simulink model "qdrdac_newphscrct"  (R2012b)
settings: Solver=ode45  StartTime=0.0  StopTime=22000  RelTol=1e-3
undefined symbols (not defined in the file or in its folder): pfb_coeff_gen_calc, sfp
libraries: xbsIndex_r4 x3696, casper_library_misc x76, xps_library x14, casper_library_delays x12, maddogLibrary x4, simulink x2
(part 9 of 37)

== system qdrdac_newphscrct/pfb_fir1 ==
  sync : Inport
  pol1_in1 : Inport  Port=2
  pol1_in2 : Inport  Port=3
  pol1_in3 : Inport  Port=4
  pol1_in4 : Inport  Port=5
  pol1_in1_coeffs : Subsystem  AncestorBlock=casper_library_pfbs/pfb_coeff_gen  mask(pfb_coeff_gen){PFBSize=9, CoeffBitWidth=18, TotalTaps=4, CoeffDistMem=off, WindowType=hamming, bram_latency=2, n_inputs=2, nput=0, fwidth=1, debug_mode=off, fan_latency=1}
      mask prompts: PFBSize "Size of PFB: (2^? pnts)"; CoeffBitWidth "Bitwidth of Coefficients:"; TotalTaps "Total Number of Taps:"; CoeffDistMem "Implement Coeff Gen in Distributed Memory"; WindowType "Windowing Function:"; bram_latency "BRAM Latency"; n_inputs "Number of Simultaneous Inputs: (2^?)"; nput "This is input number:"; fwidth "Bin Width (normal=1)"; debug_mode "Debug mode - coeffs are a [1:pfb_size*taps] ramp."; fan_latency "Fanout latency"
      mask init:
      | pfb_coeff_gen_init(gcb, ...
      |     'PFBSize', PFBSize, ...
      |     'CoeffBitWidth', CoeffBitWidth, ...
      |     'TotalTaps', TotalTaps, ...
      |     'CoeffDistMem', CoeffDistMem, ...
      |     'WindowType', WindowType, ...
      |     'bram_latency', bram_latency, ...
      |     'n_inputs', n_inputs, ...
      |     'nput', nput, ...
      |     'fwidth', fwidth, ...
      |     'fan_latency', fan_latency, ...
      |     'debug_mode', debug_mode);
      settings: AttributesFormatString=|
      | PFBSize=9, n_inputs=2,
      | taps=4, input=0
  pol1_in1_first_tap : Subsystem  AncestorBlock=casper_library_pfbs/first_tap  mask(first_tap){PFBSize=9, CoeffBitWidth=18, TotalTaps=4, BitWidthIn=12, WindowType=hamming, mult_latency=2, bram_latency=2, n_inputs=2, fwidth=1, use_hdl=on, use_embedded=off}
      mask prompts: PFBSize "Size of PFB: (2^? pnts)"; CoeffBitWidth "Bitwidth of Coefficients:"; TotalTaps "Total Number of Taps:"; BitWidthIn "Input Bitwidth:"; WindowType "Windowing Function:"; mult_latency "Mult Latency"; bram_latency "BRAM Latency"; n_inputs "Number of Simultaneous Inputs: (2^?)"; fwidth "Bit Width (normal=1)"; use_hdl "Use behavioral HDL for multlipliers"; use_embedded "Use embedded multipliers"
      mask init:
      | first_tap_init(gcb,...
      |     'PFBSize', PFBSize,...
      |     'CoeffBitWidth', CoeffBitWidth,...
      |     'TotalTaps', TotalTaps,...
      |     'BitWidthIn', BitWidthIn,...
      |     'WindowType', WindowType,...
      |     'mult_latency', mult_latency,...
      |     'bram_latency', bram_latency,...
      |     'n_inputs', n_inputs,...
      |     'fwidth', fwidth,...
      |     'use_hdl', use_hdl,...
      |     'use_embedded', use_embedded);
      settings: AttributesFormatString=taps=4
      mask TypeOptions WindowType: bartlett | barthannwin | blackman | blackmanharris | bohamwin | chebwin | flattopwin | gausswin | hamming | hann | kaiser | nuttallwin | parzenwin | rectwin | tukeywin | triang
      mask Callback use_hdl:
      | use_hdl = get_param(gcb,'use_hdl');
      | if( strcmp(use_hdl,'on')),
      |     set_param(gcb, 'use_embedded','off');
      |     set_param(gcb, 'MaskVisibilities',{'on','on','on','on','on','on','on','on','on','on','off'});
      | else,
      |     set_param(gcb, 'MaskVisibilities',{'on','on','on','on','on','on','on','on','on','on','on'});
      | end
  pol1_in1_last_tap : Subsystem  AncestorBlock=casper_library_pfbs/last_tap  mask(last_tap){TotalTaps=4, BitWidthIn=12, BitWidthOut=18, CoeffBitWidth=18, add_latency=1, mult_latency=2, quantization=Truncate, use_hdl=on, use_embedded=off}
      mask prompts: TotalTaps "Total Number of Taps:"; BitWidthIn "Input Bitwidth:"; BitWidthOut "Output Bitwidth:"; CoeffBitWidth "Coeff Bitwidth:"; add_latency "Add Latency"; mult_latency "Mult Latency"; quantization "Quantization Behavior"; use_hdl "Use behavioral HDL for multlipliers"; use_embedded "Use embedded multipliers"
      mask init:
      | last_tap_init(gcb,...
      |     'TotalTaps', TotalTaps,...
      |     'BitWidthIn', BitWidthIn,...
      |     'BitWidthOut', BitWidthOut,...
      |     'CoeffBitWidth', CoeffBitWidth,...
      |     'add_latency', add_latency,...
      |     'mult_latency', mult_latency,...
      |     'quantization', quantization,...
      |     'use_hdl', use_hdl,...
      |     'use_embedded', use_embedded);
      settings: AttributesFormatString=taps=4
      mask TypeOptions quantization: Truncate | Round  (unbiased: +/- Inf) | Round  (unbiased: Even Values)
      mask Callback use_hdl:
      | use_hdl = get_param(gcb,'use_hdl');
      | if( strcmp(use_hdl,'on')),
      |     set_param(gcb, 'use_embedded','off');
      |     set_param(gcb, 'MaskVisibilities',{'on','on','on','on','on','on','on','on','off'});
      | else,
      |     set_param(gcb, 'MaskVisibilities',{'on','on','on','on','on','on','on','on','on'});
      | end
  pol1_in1_tap2 : Subsystem  AncestorBlock=casper_library_pfbs/tap  mask(tap){mult_latency=2, coeff_width=18, coeff_frac_width=17, delay=128, data_width=12, bram_latency=2, use_hdl=on, use_embedded=off}
      mask prompts: mult_latency "Multiplier Latency"; coeff_width "Coefficient Bit Width In"; coeff_frac_width "Coefficient Fractional Bits"; delay "Data/Sync Delay"; data_width "Data Bit Width In"; bram_latency "BRAM Latency"; use_hdl "Use behavioral HDL for multlipliers"; use_embedded "Use embedded multipliers"
      mask init:
      | use_hdl = get_param(gcb,'use_hdl');
      | use_embedded = get_param(gcb,'use_embedded');
      | set_param(gcb,'LinkStatus','inactive');
      | 
      | set_param([gcb,'/Mult'],'use_embedded',use_embedded);
      | set_param([gcb,'/Mult'],'use_behavioral_HDL',use_hdl);
      | set_param([gcb,'/Mult1'],'use_embedded',use_embedded);
      | set_param([gcb,'/Mult1'],'use_behavioral_HDL',use_hdl);
      mask Callback use_hdl:
      | use_hdl = get_param(gcb,'use_hdl');
      | if( strcmp(use_hdl,'on')),
      |     set_param(gcb, 'use_embedded','off');
      |     set_param(gcb, 'MaskVisibilities',{'on','on','on','on','on','on','on','off'});
      | else,
      |     set_param(gcb, 'MaskVisibilities',{'on','on','on','on','on','on','on','on'});
      | end
  pol1_in1_tap3 : Subsystem  AncestorBlock=casper_library_pfbs/tap  mask(tap){mult_latency=2, coeff_width=18, coeff_frac_width=17, delay=128, data_width=12, bram_latency=2, use_hdl=on, use_embedded=off}
      mask prompts: mult_latency "Multiplier Latency"; coeff_width "Coefficient Bit Width In"; coeff_frac_width "Coefficient Fractional Bits"; delay "Data/Sync Delay"; data_width "Data Bit Width In"; bram_latency "BRAM Latency"; use_hdl "Use behavioral HDL for multlipliers"; use_embedded "Use embedded multipliers"
      mask init: same as qdrdac_newphscrct/pfb_fir1/pol1_in1_tap2
      mask Callback use_hdl:
      | use_hdl = get_param(gcb,'use_hdl');
      | if( strcmp(use_hdl,'on')),
      |     set_param(gcb, 'use_embedded','off');
      |     set_param(gcb, 'MaskVisibilities',{'on','on','on','on','on','on','on','off'});
      | else,
      |     set_param(gcb, 'MaskVisibilities',{'on','on','on','on','on','on','on','on'});
      | end
  pol1_in2_coeffs : Subsystem  AncestorBlock=casper_library_pfbs/pfb_coeff_gen  mask(pfb_coeff_gen){PFBSize=9, CoeffBitWidth=18, TotalTaps=4, CoeffDistMem=off, WindowType=hamming, bram_latency=2, n_inputs=2, nput=1, fwidth=1, debug_mode=off, fan_latency=1}
      mask prompts: PFBSize "Size of PFB: (2^? pnts)"; CoeffBitWidth "Bitwidth of Coefficients:"; TotalTaps "Total Number of Taps:"; CoeffDistMem "Implement Coeff Gen in Distributed Memory"; WindowType "Windowing Function:"; bram_latency "BRAM Latency"; n_inputs "Number of Simultaneous Inputs: (2^?)"; nput "This is input number:"; fwidth "Bin Width (normal=1)"; debug_mode "Debug mode - coeffs are a [1:pfb_size*taps] ramp."; fan_latency "Fanout latency"
      mask init: same as qdrdac_newphscrct/pfb_fir1/pol1_in1_coeffs
      settings: AttributesFormatString=|
      | PFBSize=9, n_inputs=2,
      | taps=4, input=1
  pol1_in2_first_tap : Subsystem  AncestorBlock=casper_library_pfbs/first_tap  mask(first_tap){PFBSize=9, CoeffBitWidth=18, TotalTaps=4, BitWidthIn=12, WindowType=hamming, mult_latency=2, bram_latency=2, n_inputs=2, fwidth=1, use_hdl=on, use_embedded=off}
      mask prompts: PFBSize "Size of PFB: (2^? pnts)"; CoeffBitWidth "Bitwidth of Coefficients:"; TotalTaps "Total Number of Taps:"; BitWidthIn "Input Bitwidth:"; WindowType "Windowing Function:"; mult_latency "Mult Latency"; bram_latency "BRAM Latency"; n_inputs "Number of Simultaneous Inputs: (2^?)"; fwidth "Bit Width (normal=1)"; use_hdl "Use behavioral HDL for multlipliers"; use_embedded "Use embedded multipliers"
      mask init: same as qdrdac_newphscrct/pfb_fir1/pol1_in1_first_tap
      settings: AttributesFormatString=taps=4
      mask TypeOptions WindowType: bartlett | barthannwin | blackman | blackmanharris | bohamwin | chebwin | flattopwin | gausswin | hamming | hann | kaiser | nuttallwin | parzenwin | rectwin | tukeywin | triang
      mask Callback use_hdl:
      | use_hdl = get_param(gcb,'use_hdl');
      | if( strcmp(use_hdl,'on')),
      |     set_param(gcb, 'use_embedded','off');
      |     set_param(gcb, 'MaskVisibilities',{'on','on','on','on','on','on','on','on','on','on','off'});
      | else,
      |     set_param(gcb, 'MaskVisibilities',{'on','on','on','on','on','on','on','on','on','on','on'});
      | end
  pol1_in2_last_tap : Subsystem  AncestorBlock=casper_library_pfbs/last_tap  mask(last_tap){TotalTaps=4, BitWidthIn=12, BitWidthOut=18, CoeffBitWidth=18, add_latency=1, mult_latency=2, quantization=Truncate, use_hdl=on, use_embedded=off}
      mask prompts: TotalTaps "Total Number of Taps:"; BitWidthIn "Input Bitwidth:"; BitWidthOut "Output Bitwidth:"; CoeffBitWidth "Coeff Bitwidth:"; add_latency "Add Latency"; mult_latency "Mult Latency"; quantization "Quantization Behavior"; use_hdl "Use behavioral HDL for multlipliers"; use_embedded "Use embedded multipliers"
      mask init: same as qdrdac_newphscrct/pfb_fir1/pol1_in1_last_tap
      settings: AttributesFormatString=taps=4
      mask TypeOptions quantization: Truncate | Round  (unbiased: +/- Inf) | Round  (unbiased: Even Values)
      mask Callback use_hdl:
      | use_hdl = get_param(gcb,'use_hdl');
      | if( strcmp(use_hdl,'on')),
      |     set_param(gcb, 'use_embedded','off');
      |     set_param(gcb, 'MaskVisibilities',{'on','on','on','on','on','on','on','on','off'});
      | else,
      |     set_param(gcb, 'MaskVisibilities',{'on','on','on','on','on','on','on','on','on'});
      | end
  pol1_in2_tap2 : Subsystem  AncestorBlock=casper_library_pfbs/tap  mask(tap){mult_latency=2, coeff_width=18, coeff_frac_width=17, delay=128, data_width=12, bram_latency=2, use_hdl=on, use_embedded=off}
      mask prompts: mult_latency "Multiplier Latency"; coeff_width "Coefficient Bit Width In"; coeff_frac_width "Coefficient Fractional Bits"; delay "Data/Sync Delay"; data_width "Data Bit Width In"; bram_latency "BRAM Latency"; use_hdl "Use behavioral HDL for multlipliers"; use_embedded "Use embedded multipliers"
      mask init: same as qdrdac_newphscrct/pfb_fir1/pol1_in1_tap2
      mask Callback use_hdl:
      | use_hdl = get_param(gcb,'use_hdl');
      | if( strcmp(use_hdl,'on')),
      |     set_param(gcb, 'use_embedded','off');
      |     set_param(gcb, 'MaskVisibilities',{'on','on','on','on','on','on','on','off'});
      | else,
      |     set_param(gcb, 'MaskVisibilities',{'on','on','on','on','on','on','on','on'});
      | end
  pol1_in2_tap3 : Subsystem  AncestorBlock=casper_library_pfbs/tap  mask(tap){mult_latency=2, coeff_width=18, coeff_frac_width=17, delay=128, data_width=12, bram_latency=2, use_hdl=on, use_embedded=off}
      mask prompts: mult_latency "Multiplier Latency"; coeff_width "Coefficient Bit Width In"; coeff_frac_width "Coefficient Fractional Bits"; delay "Data/Sync Delay"; data_width "Data Bit Width In"; bram_latency "BRAM Latency"; use_hdl "Use behavioral HDL for multlipliers"; use_embedded "Use embedded multipliers"
      mask init: same as qdrdac_newphscrct/pfb_fir1/pol1_in1_tap2
      mask Callback use_hdl:
      | use_hdl = get_param(gcb,'use_hdl');
      | if( strcmp(use_hdl,'on')),
      |     set_param(gcb, 'use_embedded','off');
      |     set_param(gcb, 'MaskVisibilities',{'on','on','on','on','on','on','on','off'});
      | else,
      |     set_param(gcb, 'MaskVisibilities',{'on','on','on','on','on','on','on','on'});
      | end
  pol1_in3_coeffs : Subsystem  AncestorBlock=casper_library_pfbs/pfb_coeff_gen  mask(pfb_coeff_gen){PFBSize=9, CoeffBitWidth=18, TotalTaps=4, CoeffDistMem=off, WindowType=hamming, bram_latency=2, n_inputs=2, nput=2, fwidth=1, debug_mode=off, fan_latency=1}
      mask prompts: PFBSize "Size of PFB: (2^? pnts)"; CoeffBitWidth "Bitwidth of Coefficients:"; TotalTaps "Total Number of Taps:"; CoeffDistMem "Implement Coeff Gen in Distributed Memory"; WindowType "Windowing Function:"; bram_latency "BRAM Latency"; n_inputs "Number of Simultaneous Inputs: (2^?)"; nput "This is input number:"; fwidth "Bin Width (normal=1)"; debug_mode "Debug mode - coeffs are a [1:pfb_size*taps] ramp."; fan_latency "Fanout latency"
      mask init: same as qdrdac_newphscrct/pfb_fir1/pol1_in1_coeffs
      settings: AttributesFormatString=|
      | PFBSize=9, n_inputs=2,
      | taps=4, input=2
  pol1_in3_first_tap : Subsystem  AncestorBlock=casper_library_pfbs/first_tap  mask(first_tap){PFBSize=9, CoeffBitWidth=18, TotalTaps=4, BitWidthIn=12, WindowType=hamming, mult_latency=2, bram_latency=2, n_inputs=2, fwidth=1, use_hdl=on, use_embedded=off}
      mask prompts: PFBSize "Size of PFB: (2^? pnts)"; CoeffBitWidth "Bitwidth of Coefficients:"; TotalTaps "Total Number of Taps:"; BitWidthIn "Input Bitwidth:"; WindowType "Windowing Function:"; mult_latency "Mult Latency"; bram_latency "BRAM Latency"; n_inputs "Number of Simultaneous Inputs: (2^?)"; fwidth "Bit Width (normal=1)"; use_hdl "Use behavioral HDL for multlipliers"; use_embedded "Use embedded multipliers"
      mask init: same as qdrdac_newphscrct/pfb_fir1/pol1_in1_first_tap
      settings: AttributesFormatString=taps=4
      mask TypeOptions WindowType: bartlett | barthannwin | blackman | blackmanharris | bohamwin | chebwin | flattopwin | gausswin | hamming | hann | kaiser | nuttallwin | parzenwin | rectwin | tukeywin | triang
      mask Callback use_hdl:
      | use_hdl = get_param(gcb,'use_hdl');
      | if( strcmp(use_hdl,'on')),
      |     set_param(gcb, 'use_embedded','off');
      |     set_param(gcb, 'MaskVisibilities',{'on','on','on','on','on','on','on','on','on','on','off'});
      | else,
      |     set_param(gcb, 'MaskVisibilities',{'on','on','on','on','on','on','on','on','on','on','on'});
      | end
  pol1_in3_last_tap : Subsystem  AncestorBlock=casper_library_pfbs/last_tap  mask(last_tap){TotalTaps=4, BitWidthIn=12, BitWidthOut=18, CoeffBitWidth=18, add_latency=1, mult_latency=2, quantization=Truncate, use_hdl=on, use_embedded=off}
      mask prompts: TotalTaps "Total Number of Taps:"; BitWidthIn "Input Bitwidth:"; BitWidthOut "Output Bitwidth:"; CoeffBitWidth "Coeff Bitwidth:"; add_latency "Add Latency"; mult_latency "Mult Latency"; quantization "Quantization Behavior"; use_hdl "Use behavioral HDL for multlipliers"; use_embedded "Use embedded multipliers"
      mask init: same as qdrdac_newphscrct/pfb_fir1/pol1_in1_last_tap
      settings: AttributesFormatString=taps=4
      mask TypeOptions quantization: Truncate | Round  (unbiased: +/- Inf) | Round  (unbiased: Even Values)
      mask Callback use_hdl:
      | use_hdl = get_param(gcb,'use_hdl');
      | if( strcmp(use_hdl,'on')),
      |     set_param(gcb, 'use_embedded','off');
      |     set_param(gcb, 'MaskVisibilities',{'on','on','on','on','on','on','on','on','off'});
      | else,
      |     set_param(gcb, 'MaskVisibilities',{'on','on','on','on','on','on','on','on','on'});
      | end
  pol1_in3_tap2 : Subsystem  AncestorBlock=casper_library_pfbs/tap  mask(tap){mult_latency=2, coeff_width=18, coeff_frac_width=17, delay=128, data_width=12, bram_latency=2, use_hdl=on, use_embedded=off}
      mask prompts: mult_latency "Multiplier Latency"; coeff_width "Coefficient Bit Width In"; coeff_frac_width "Coefficient Fractional Bits"; delay "Data/Sync Delay"; data_width "Data Bit Width In"; bram_latency "BRAM Latency"; use_hdl "Use behavioral HDL for multlipliers"; use_embedded "Use embedded multipliers"
      mask init: same as qdrdac_newphscrct/pfb_fir1/pol1_in1_tap2
      mask Callback use_hdl:
      | use_hdl = get_param(gcb,'use_hdl');
      | if( strcmp(use_hdl,'on')),
      |     set_param(gcb, 'use_embedded','off');
      |     set_param(gcb, 'MaskVisibilities',{'on','on','on','on','on','on','on','off'});
      | else,
      |     set_param(gcb, 'MaskVisibilities',{'on','on','on','on','on','on','on','on'});
      | end
  pol1_in3_tap3 : Subsystem  AncestorBlock=casper_library_pfbs/tap  mask(tap){mult_latency=2, coeff_width=18, coeff_frac_width=17, delay=128, data_width=12, bram_latency=2, use_hdl=on, use_embedded=off}
      mask prompts: mult_latency "Multiplier Latency"; coeff_width "Coefficient Bit Width In"; coeff_frac_width "Coefficient Fractional Bits"; delay "Data/Sync Delay"; data_width "Data Bit Width In"; bram_latency "BRAM Latency"; use_hdl "Use behavioral HDL for multlipliers"; use_embedded "Use embedded multipliers"
      mask init: same as qdrdac_newphscrct/pfb_fir1/pol1_in1_tap2
      mask Callback use_hdl:
      | use_hdl = get_param(gcb,'use_hdl');
      | if( strcmp(use_hdl,'on')),
      |     set_param(gcb, 'use_embedded','off');
      |     set_param(gcb, 'MaskVisibilities',{'on','on','on','on','on','on','on','off'});
      | else,
      |     set_param(gcb, 'MaskVisibilities',{'on','on','on','on','on','on','on','on'});
      | end
  pol1_in4_coeffs : Subsystem  AncestorBlock=casper_library_pfbs/pfb_coeff_gen  mask(pfb_coeff_gen){PFBSize=9, CoeffBitWidth=18, TotalTaps=4, CoeffDistMem=off, WindowType=hamming, bram_latency=2, n_inputs=2, nput=3, fwidth=1, debug_mode=off, fan_latency=1}
      mask prompts: PFBSize "Size of PFB: (2^? pnts)"; CoeffBitWidth "Bitwidth of Coefficients:"; TotalTaps "Total Number of Taps:"; CoeffDistMem "Implement Coeff Gen in Distributed Memory"; WindowType "Windowing Function:"; bram_latency "BRAM Latency"; n_inputs "Number of Simultaneous Inputs: (2^?)"; nput "This is input number:"; fwidth "Bin Width (normal=1)"; debug_mode "Debug mode - coeffs are a [1:pfb_size*taps] ramp."; fan_latency "Fanout latency"
      mask init: same as qdrdac_newphscrct/pfb_fir1/pol1_in1_coeffs
      settings: AttributesFormatString=|
      | PFBSize=9, n_inputs=2,
      | taps=4, input=3
  pol1_in4_first_tap : Subsystem  AncestorBlock=casper_library_pfbs/first_tap  mask(first_tap){PFBSize=9, CoeffBitWidth=18, TotalTaps=4, BitWidthIn=12, WindowType=hamming, mult_latency=2, bram_latency=2, n_inputs=2, fwidth=1, use_hdl=on, use_embedded=off}
      mask prompts: PFBSize "Size of PFB: (2^? pnts)"; CoeffBitWidth "Bitwidth of Coefficients:"; TotalTaps "Total Number of Taps:"; BitWidthIn "Input Bitwidth:"; WindowType "Windowing Function:"; mult_latency "Mult Latency"; bram_latency "BRAM Latency"; n_inputs "Number of Simultaneous Inputs: (2^?)"; fwidth "Bit Width (normal=1)"; use_hdl "Use behavioral HDL for multlipliers"; use_embedded "Use embedded multipliers"
      mask init: same as qdrdac_newphscrct/pfb_fir1/pol1_in1_first_tap
      settings: AttributesFormatString=taps=4
      mask TypeOptions WindowType: bartlett | barthannwin | blackman | blackmanharris | bohamwin | chebwin | flattopwin | gausswin | hamming | hann | kaiser | nuttallwin | parzenwin | rectwin | tukeywin | triang
      mask Callback use_hdl:
      | use_hdl = get_param(gcb,'use_hdl');
      | if( strcmp(use_hdl,'on')),
      |     set_param(gcb, 'use_embedded','off');
      |     set_param(gcb, 'MaskVisibilities',{'on','on','on','on','on','on','on','on','on','on','off'});
      | else,
      |     set_param(gcb, 'MaskVisibilities',{'on','on','on','on','on','on','on','on','on','on','on'});
      | end
  pol1_in4_last_tap : Subsystem  AncestorBlock=casper_library_pfbs/last_tap  mask(last_tap){TotalTaps=4, BitWidthIn=12, BitWidthOut=18, CoeffBitWidth=18, add_latency=1, mult_latency=2, quantization=Truncate, use_hdl=on, use_embedded=off}
      mask prompts: TotalTaps "Total Number of Taps:"; BitWidthIn "Input Bitwidth:"; BitWidthOut "Output Bitwidth:"; CoeffBitWidth "Coeff Bitwidth:"; add_latency "Add Latency"; mult_latency "Mult Latency"; quantization "Quantization Behavior"; use_hdl "Use behavioral HDL for multlipliers"; use_embedded "Use embedded multipliers"
      mask init: same as qdrdac_newphscrct/pfb_fir1/pol1_in1_last_tap
      settings: AttributesFormatString=taps=4
      mask TypeOptions quantization: Truncate | Round  (unbiased: +/- Inf) | Round  (unbiased: Even Values)
      mask Callback use_hdl:
      | use_hdl = get_param(gcb,'use_hdl');
      | if( strcmp(use_hdl,'on')),
      |     set_param(gcb, 'use_embedded','off');
      |     set_param(gcb, 'MaskVisibilities',{'on','on','on','on','on','on','on','on','off'});
      | else,
      |     set_param(gcb, 'MaskVisibilities',{'on','on','on','on','on','on','on','on','on'});
      | end
  pol1_in4_tap2 : Subsystem  AncestorBlock=casper_library_pfbs/tap  mask(tap){mult_latency=2, coeff_width=18, coeff_frac_width=17, delay=128, data_width=12, bram_latency=2, use_hdl=on, use_embedded=off}
      mask prompts: mult_latency "Multiplier Latency"; coeff_width "Coefficient Bit Width In"; coeff_frac_width "Coefficient Fractional Bits"; delay "Data/Sync Delay"; data_width "Data Bit Width In"; bram_latency "BRAM Latency"; use_hdl "Use behavioral HDL for multlipliers"; use_embedded "Use embedded multipliers"
      mask init: same as qdrdac_newphscrct/pfb_fir1/pol1_in1_tap2
      mask Callback use_hdl:
      | use_hdl = get_param(gcb,'use_hdl');
      | if( strcmp(use_hdl,'on')),
      |     set_param(gcb, 'use_embedded','off');
      |     set_param(gcb, 'MaskVisibilities',{'on','on','on','on','on','on','on','off'});
      | else,
      |     set_param(gcb, 'MaskVisibilities',{'on','on','on','on','on','on','on','on'});
      | end
  pol1_in4_tap3 : Subsystem  AncestorBlock=casper_library_pfbs/tap  mask(tap){mult_latency=2, coeff_width=18, coeff_frac_width=17, delay=128, data_width=12, bram_latency=2, use_hdl=on, use_embedded=off}
      mask prompts: mult_latency "Multiplier Latency"; coeff_width "Coefficient Bit Width In"; coeff_frac_width "Coefficient Fractional Bits"; delay "Data/Sync Delay"; data_width "Data Bit Width In"; bram_latency "BRAM Latency"; use_hdl "Use behavioral HDL for multlipliers"; use_embedded "Use embedded multipliers"
      mask init: same as qdrdac_newphscrct/pfb_fir1/pol1_in1_tap2
      mask Callback use_hdl:
      | use_hdl = get_param(gcb,'use_hdl');
      | if( strcmp(use_hdl,'on')),
      |     set_param(gcb, 'use_embedded','off');
      |     set_param(gcb, 'MaskVisibilities',{'on','on','on','on','on','on','on','off'});
      | else,
      |     set_param(gcb, 'MaskVisibilities',{'on','on','on','on','on','on','on','on'});
      | end
  sync_out : Outport
  pol1_out1 : Outport  Port=2
  pol1_out2 : Outport  Port=3
  pol1_out3 : Outport  Port=4
  pol1_out4 : Outport  Port=5
  wires:
  pol1_in1/1 -> pol1_in1_coeffs/1(din)
  sync/1 -> pol1_in1_coeffs/2(sync), pol1_in2_coeffs/2(sync), pol1_in3_coeffs/2(sync), pol1_in4_coeffs/2(sync)
  pol1_in1_coeffs/1(dout) -> pol1_in1_first_tap/1(din)
  pol1_in1_coeffs/2(sync_out) -> pol1_in1_first_tap/2(sync), pol1_in2_first_tap/2(sync), pol1_in3_first_tap/2(sync), pol1_in4_first_tap/2(sync)
  pol1_in1_coeffs/3(coeff) -> pol1_in1_first_tap/3(coeffs)
  pol1_in1_first_tap/1(dout) -> pol1_in1_tap2/1(din)
  pol1_in1_first_tap/2(sync_out) -> pol1_in1_tap2/2(sync)
  pol1_in1_first_tap/3(coeff_out) -> pol1_in1_tap2/3(coeff)
  pol1_in1_first_tap/4(taps_out) -> pol1_in1_tap2/4(taps)
  pol1_in1_tap2/1(dout) -> pol1_in1_tap3/1(din)
  pol1_in1_tap2/2(sync_out) -> pol1_in1_tap3/2(sync)
  pol1_in1_tap2/3(coeff_out) -> pol1_in1_tap3/3(coeff)
  pol1_in1_tap2/4(taps_out) -> pol1_in1_tap3/4(taps)
  pol1_in1_tap3/1(dout) -> pol1_in1_last_tap/1(din)
  pol1_in1_tap3/2(sync_out) -> pol1_in1_last_tap/2(sync)
  pol1_in1_tap3/3(coeff_out) -> pol1_in1_last_tap/3(coeff)
  pol1_in1_tap3/4(taps_out) -> pol1_in1_last_tap/4(taps)
  pol1_in1_last_tap/1(dout) -> pol1_out1/1
  pol1_in1_last_tap/2(sync_out) -> sync_out/1
  pol1_in2/1 -> pol1_in2_coeffs/1(din)
  pol1_in2_coeffs/1(dout) -> pol1_in2_first_tap/1(din)
  pol1_in2_coeffs/3(coeff) -> pol1_in2_first_tap/3(coeffs)
  pol1_in2_first_tap/1(dout) -> pol1_in2_tap2/1(din)
  pol1_in2_first_tap/2(sync_out) -> pol1_in2_tap2/2(sync)
  pol1_in2_first_tap/3(coeff_out) -> pol1_in2_tap2/3(coeff)
  pol1_in2_first_tap/4(taps_out) -> pol1_in2_tap2/4(taps)
  pol1_in2_tap2/1(dout) -> pol1_in2_tap3/1(din)
  pol1_in2_tap2/2(sync_out) -> pol1_in2_tap3/2(sync)
  pol1_in2_tap2/3(coeff_out) -> pol1_in2_tap3/3(coeff)
  pol1_in2_tap2/4(taps_out) -> pol1_in2_tap3/4(taps)
  pol1_in2_tap3/1(dout) -> pol1_in2_last_tap/1(din)
  pol1_in2_tap3/2(sync_out) -> pol1_in2_last_tap/2(sync)
  pol1_in2_tap3/3(coeff_out) -> pol1_in2_last_tap/3(coeff)
  pol1_in2_tap3/4(taps_out) -> pol1_in2_last_tap/4(taps)
  pol1_in2_last_tap/1(dout) -> pol1_out2/1
  pol1_in3/1 -> pol1_in3_coeffs/1(din)
  pol1_in3_coeffs/1(dout) -> pol1_in3_first_tap/1(din)
  pol1_in3_coeffs/3(coeff) -> pol1_in3_first_tap/3(coeffs)
  pol1_in3_first_tap/1(dout) -> pol1_in3_tap2/1(din)
  pol1_in3_first_tap/2(sync_out) -> pol1_in3_tap2/2(sync)
  pol1_in3_first_tap/3(coeff_out) -> pol1_in3_tap2/3(coeff)
  pol1_in3_first_tap/4(taps_out) -> pol1_in3_tap2/4(taps)
  pol1_in3_tap2/1(dout) -> pol1_in3_tap3/1(din)
  pol1_in3_tap2/2(sync_out) -> pol1_in3_tap3/2(sync)
  pol1_in3_tap2/3(coeff_out) -> pol1_in3_tap3/3(coeff)
  pol1_in3_tap2/4(taps_out) -> pol1_in3_tap3/4(taps)
  pol1_in3_tap3/1(dout) -> pol1_in3_last_tap/1(din)
  pol1_in3_tap3/2(sync_out) -> pol1_in3_last_tap/2(sync)
  pol1_in3_tap3/3(coeff_out) -> pol1_in3_last_tap/3(coeff)
  pol1_in3_tap3/4(taps_out) -> pol1_in3_last_tap/4(taps)
  pol1_in3_last_tap/1(dout) -> pol1_out3/1
  pol1_in4/1 -> pol1_in4_coeffs/1(din)
  pol1_in4_coeffs/1(dout) -> pol1_in4_first_tap/1(din)
  pol1_in4_coeffs/3(coeff) -> pol1_in4_first_tap/3(coeffs)
  pol1_in4_first_tap/1(dout) -> pol1_in4_tap2/1(din)
  pol1_in4_first_tap/2(sync_out) -> pol1_in4_tap2/2(sync)
  pol1_in4_first_tap/3(coeff_out) -> pol1_in4_tap2/3(coeff)
  pol1_in4_first_tap/4(taps_out) -> pol1_in4_tap2/4(taps)
  pol1_in4_tap2/1(dout) -> pol1_in4_tap3/1(din)
  pol1_in4_tap2/2(sync_out) -> pol1_in4_tap3/2(sync)
  pol1_in4_tap2/3(coeff_out) -> pol1_in4_tap3/3(coeff)
  pol1_in4_tap2/4(taps_out) -> pol1_in4_tap3/4(taps)
  pol1_in4_tap3/1(dout) -> pol1_in4_last_tap/1(din)
  pol1_in4_tap3/2(sync_out) -> pol1_in4_last_tap/2(sync)
  pol1_in4_tap3/3(coeff_out) -> pol1_in4_last_tap/3(coeff)
  pol1_in4_tap3/4(taps_out) -> pol1_in4_last_tap/4(taps)
  pol1_in4_last_tap/1(dout) -> pol1_out4/1

== system qdrdac_newphscrct/readFifoSize ==
  sim_1 : Inport
  io_delay : xbsIndex_r4/Delay  rst=off  infoeditControl=Selection of Reset will increase slice count due to use of real FFs and instead of SRLs  en=off  latency=0  dbl_ovrd=off  reg_retiming=on  block_type=delay
  qdrdac_readFifoSize_user_data_out : xbsIndex_r4/Gateway In  gui_display_data_type=Fixed-point  arith_type=Unsigned  n_bits=32  bin_pt=0  preci_type=Single  exp_width=8  frac_width=24  quantization="Round  (unbiased: +/- Inf)"  overflow=Saturate  period=1  dbl_ovrd=off  timing_constraint=None  locs_specified=off  LOCs={}  UseAsADC=off  ADCChannel='1'  inherit_from_input=off  hdl_port=on  block_type=gatewayin
  reint1 : xbsIndex_r4/Reinterpret  force_arith_type=on  arith_type=Unsigned  force_bin_pt=on  bin_pt=0  block_type=reinterpret
  slice_reg : xbsIndex_r4/Slice  nbits=8  boolean_output=off  mode=Lower Bit Location + Width  bit1=0  base1=MSB of Input  bit0=0  base0=LSB of Input  dbl_ovrd=off  block_type=slice
  in_reg : Outport
  wires:
  qdrdac_readFifoSize_user_data_out/1 -> io_delay/1
  sim_1/1 -> qdrdac_readFifoSize_user_data_out/1
  io_delay/1 -> slice_reg/1
  slice_reg/1 -> reint1/1
  reint1/1 -> in_reg/1

== system qdrdac_newphscrct/rect2polarV1 ==
  dvalid : Inport
  cmplx : Inport  Port=2
  chan : Inport  Port=3
  "CORDIC 5.0 " : xbsIndex_r4/CORDIC 5.0   functional_selection=Translate  architectural_configuration=Parallel  pipelining_mode=Maximum  data_format=SignedFraction  phase_format=Scaled_Radians  input_width=18  output_width=18  round_mode=Truncate  iterations=0  precision=0  compensation_scaling=Embedded_Multiplier  coarse_rotation=on  aclken=off  aresetn=off  out_tready=off  cartesian_has_tuser=off  cartesian_has_tlast=off  cartesian_tuser_width=1  phase_has_tuser=off  phase_has_tlast=off  phase_tuser_width=1  out_tlast_behv=Null  flow_control=NonBlocking  optimize_goal=Resources  trim_axipin_name=on  ip_name=CORDIC  ip_version=5.0  dsptool_ready=true  ipcore_usecache=true  ipcore_useipmodelcache=true  wrapper_available=true  port_translation_map={ 'aclken' => 'en', 'aresetn' => 'rst' }  block_type=cordic_v5_0
      settings: infoedit=CORDIC 5.0
  Delay : xbsIndex_r4/Delay  rst=off  infoeditControl=Selection of Reset will increase slice count due to use of real FFs and instead of SRLs  en=off  latency=25  dbl_ovrd=off  reg_retiming=off  block_type=delay
  c_to_ri3 : casper_library_misc/c_to_ri  n_bits=18  bin_pt=16
      settings: AttributesFormatString=18_16 r/i
  ri_to_c : casper_library_misc/ri_to_c
  dvalidout : Outport
  pol : Outport  Port=2
  chandly : Outport  Port=3
  wires:
  cmplx/1 -> c_to_ri3/1
  c_to_ri3/2 -> "CORDIC 5.0 "/2
  "CORDIC 5.0 "/2 -> ri_to_c/2
  "CORDIC 5.0 "/1 -> dvalidout/1
  ri_to_c/1 -> pol/1
  chan/1 -> Delay/1
  dvalid/1 -> "CORDIC 5.0 "/1
  "CORDIC 5.0 "/3 -> ri_to_c/1
  Delay/1 -> chandly/1
  c_to_ri3/1 -> "CORDIC 5.0 "/3

== system qdrdac_newphscrct/rect2polarV2 ==
  dvalid : Inport
  cmplx : Inport  Port=2
  chan : Inport  Port=3
  "CORDIC 5.0 " : xbsIndex_r4/CORDIC 5.0   functional_selection=Translate  architectural_configuration=Parallel  pipelining_mode=Maximum  data_format=SignedFraction  phase_format=Scaled_Radians  input_width=18  output_width=18  round_mode=Truncate  iterations=0  precision=0  compensation_scaling=Embedded_Multiplier  coarse_rotation=on  aclken=off  aresetn=off  out_tready=off  cartesian_has_tuser=off  cartesian_has_tlast=off  cartesian_tuser_width=1  phase_has_tuser=off  phase_has_tlast=off  phase_tuser_width=1  out_tlast_behv=Null  flow_control=NonBlocking  optimize_goal=Resources  trim_axipin_name=on  ip_name=CORDIC  ip_version=5.0  dsptool_ready=true  ipcore_usecache=true  ipcore_useipmodelcache=true  wrapper_available=true  port_translation_map={ 'aclken' => 'en', 'aresetn' => 'rst' }  block_type=cordic_v5_0
      settings: infoedit=CORDIC 5.0
  Delay : xbsIndex_r4/Delay  rst=off  infoeditControl=Selection of Reset will increase slice count due to use of real FFs and instead of SRLs  en=off  latency=25  dbl_ovrd=off  reg_retiming=off  block_type=delay
  c_to_ri3 : casper_library_misc/c_to_ri  n_bits=18  bin_pt=16
      settings: AttributesFormatString=18_16 r/i
  ri_to_c : casper_library_misc/ri_to_c
  dvalidout : Outport
  pol : Outport  Port=2
  chandly : Outport  Port=3
  wires:
  cmplx/1 -> c_to_ri3/1
  c_to_ri3/2 -> "CORDIC 5.0 "/2
  "CORDIC 5.0 "/2 -> ri_to_c/2
  "CORDIC 5.0 "/1 -> dvalidout/1
  ri_to_c/1 -> pol/1
  chan/1 -> Delay/1
  dvalid/1 -> "CORDIC 5.0 "/1
  "CORDIC 5.0 "/3 -> ri_to_c/1
  Delay/1 -> chandly/1
  c_to_ri3/1 -> "CORDIC 5.0 "/3

== system qdrdac_newphscrct/rect2polarV3 ==
  dvalid : Inport
  cmplx : Inport  Port=2
  chan : Inport  Port=3
  "CORDIC 5.0 " : xbsIndex_r4/CORDIC 5.0   functional_selection=Translate  architectural_configuration=Parallel  pipelining_mode=Maximum  data_format=SignedFraction  phase_format=Scaled_Radians  input_width=18  output_width=18  round_mode=Truncate  iterations=0  precision=0  compensation_scaling=Embedded_Multiplier  coarse_rotation=on  aclken=off  aresetn=off  out_tready=off  cartesian_has_tuser=off  cartesian_has_tlast=off  cartesian_tuser_width=1  phase_has_tuser=off  phase_has_tlast=off  phase_tuser_width=1  out_tlast_behv=Null  flow_control=NonBlocking  optimize_goal=Resources  trim_axipin_name=on  ip_name=CORDIC  ip_version=5.0  dsptool_ready=true  ipcore_usecache=true  ipcore_useipmodelcache=true  wrapper_available=true  port_translation_map={ 'aclken' => 'en', 'aresetn' => 'rst' }  block_type=cordic_v5_0
      settings: infoedit=CORDIC 5.0
  Delay : xbsIndex_r4/Delay  rst=off  infoeditControl=Selection of Reset will increase slice count due to use of real FFs and instead of SRLs  en=off  latency=25  dbl_ovrd=off  reg_retiming=off  block_type=delay
  c_to_ri3 : casper_library_misc/c_to_ri  n_bits=18  bin_pt=16
      settings: AttributesFormatString=18_16 r/i
  ri_to_c : casper_library_misc/ri_to_c
  dvalidout : Outport
  pol : Outport  Port=2
  chandly : Outport  Port=3
  wires:
  cmplx/1 -> c_to_ri3/1
  c_to_ri3/2 -> "CORDIC 5.0 "/2
  "CORDIC 5.0 "/2 -> ri_to_c/2
  "CORDIC 5.0 "/1 -> dvalidout/1
  ri_to_c/1 -> pol/1
  chan/1 -> Delay/1
  dvalid/1 -> "CORDIC 5.0 "/1
  "CORDIC 5.0 "/3 -> ri_to_c/1
  Delay/1 -> chandly/1
  c_to_ri3/1 -> "CORDIC 5.0 "/3

== system qdrdac_newphscrct/rect2polarV5 ==
  note: 18/18 data. phase and mag
      | phase is the im. part
  dvalid : Inport
  cmplx : Inport  Port=2
  chan : Inport  Port=3
  "CORDIC 5.0 " : xbsIndex_r4/CORDIC 5.0   functional_selection=Translate  architectural_configuration=Parallel  pipelining_mode=Maximum  data_format=SignedFraction  phase_format=Scaled_Radians  input_width=18  output_width=18  round_mode=Truncate  iterations=0  precision=0  compensation_scaling=Embedded_Multiplier  coarse_rotation=on  aclken=off  aresetn=off  out_tready=off  cartesian_has_tuser=off  cartesian_has_tlast=off  cartesian_tuser_width=1  phase_has_tuser=off  phase_has_tlast=off  phase_tuser_width=1  out_tlast_behv=Null  flow_control=NonBlocking  optimize_goal=Resources  trim_axipin_name=on  ip_name=CORDIC  ip_version=5.0  dsptool_ready=true  ipcore_usecache=true  ipcore_useipmodelcache=true  wrapper_available=true  port_translation_map={ 'aclken' => 'en', 'aresetn' => 'rst' }  block_type=cordic_v5_0
      settings: infoedit=CORDIC 5.0
  Delay : xbsIndex_r4/Delay  rst=off  infoeditControl=Selection of Reset will increase slice count due to use of real FFs and instead of SRLs  en=off  latency=25  dbl_ovrd=off  reg_retiming=off  block_type=delay
  c_to_ri3 : casper_library_misc/c_to_ri  n_bits=18  bin_pt=16
      settings: AttributesFormatString=18_16 r/i
  ri_to_c : casper_library_misc/ri_to_c
  dvalidout : Outport
  pol : Outport  Port=2
  chandly : Outport  Port=3
  wires:
  cmplx/1 -> c_to_ri3/1
  "CORDIC 5.0 "/2 -> ri_to_c/2
  "CORDIC 5.0 "/1 -> dvalidout/1
  ri_to_c/1 -> pol/1
  chan/1 -> Delay/1
  dvalid/1 -> "CORDIC 5.0 "/1
  "CORDIC 5.0 "/3 -> ri_to_c/1
  Delay/1 -> chandly/1
  c_to_ri3/1 -> "CORDIC 5.0 "/3
  c_to_ri3/2 -> "CORDIC 5.0 "/2

== system qdrdac_newphscrct/roachscope ==
  In1 : Inport
  In2 : Inport  Port=2
  In3 : Inport  Port=3
  In4 : Inport  Port=4
  In5 : Inport  Port=5
  In6 : Inport  Port=6
  In7 : Inport  Port=7
  In8 : Inport  Port=8
  Constant : xbsIndex_r4/Constant  const=1  gui_display_data_type=Boolean  arith_type=Boolean  n_bits=16  bin_pt=14  preci_type=Single  exp_width=8  frac_width=24  explicit_period=on  period=1  equ=P=C  opselect=C  inp2=PCIN>>17  opr=+  inp1=P  carry=CIN  dbl_ovrd=off  block_type=constant
  Constant3 : Constant  Value=4
  Mux : xbsIndex_r4/Mux  inputs=8  en=off  latency=0  precision=User Defined  arith_type=Unsigned  n_bits=16  bin_pt=0  quantization=Truncate  overflow=Wrap  dbl_ovrd=off  block_type=mux
  b3_0_ : xbsIndex_r4/Slice  nbits=3  boolean_output=off  mode=Lower Bit Location + Width  bit1=0  base1=MSB of Input  bit0=0  base0=LSB of Input  dbl_ovrd=off  block_type=slice
  inputsel : Subsystem  Tag=xps:sw_reg  AncestorBlock=xps_library/software register  mask(swreg){mode=one value, io_dir=From Processor, io_delay=0, sample_period=1, names=reg, bitwidths=16, arith_types=0, bin_pts=0, sim_port=on, show_format=off}
      mask prompts: io_dir "I/O direction"; io_delay "I/O delay"; sample_period "Sample period"; names "Name:"; bitwidths "Bitwidth:"; arith_types "Type (ufix=0, fix=1, bool=2):"; bin_pts "Binary pt:"; sim_port "Provide sim input/output?"; show_format "Print format string?"
      mask init:
      | swreg_init(gcb)
      settings: AttributesFormatString=1input
      mask TypeOptions mode: one value | fields of equal size | fields of arbitrary size
      mask Callback mode: swreg_cb(gcb);
      mask TypeOptions io_dir: To Processor | From Processor
      mask Callback io_dir:
      | mask_enables = get_param(gcb, 'MaskEnables');
      | mask_names = get_param(gcb, 'MaskNames');
      | if strcmp(get_param(gcb, 'io_dir'), 'To Processor'),
      |     mask_enables{ismember(mask_names, 'sample_period')} = 'off';
      | else
      |     mask_enables{ismember(mask_names, 'sample_period')} = 'on';
      | end
      | set_param(gcb, 'MaskEnables', mask_enables);
      mask Callback bitwidths:
      | swreg_maskcheck(gcb);
      | % blk = gcb;
      | % mode = get_param(blk, 'mode');
      | % current_widths = eval(get_param(blk, 'bitwidths'));
      | % if (strcmp(mode, 'one value') || strcmp(mode, 'fields of equal size')) && (length(current_widths) > 1),
      | %     error('Only one width may be specified for this mode.');
      | % elseif strcmp(mode, 'fields of arbitrary size')
      | %     current_names = textscan(strtrim(strrep(strrep(get_param(blk, 'names'), ']', ''), '[', '')), '%s');
      | %     current_names = current_names{1};
      | %     numios = length(current_names);
      | %     if length(current_widths) ~= numios,
      | %         error('%d field names specified, but %d widths?', numios, length(current_widths));
      | %     end
      | % end
      | % total_width = 0;
      | % for ctr = 1 : length(current_widths),
      | %     total_width = total_width + current_widths(ctr);
      | % end
      | % if total_width > 32,
      | %     error('Total width must be 32 or less, set to %d.', total_width);
      | % end
      mask Callback arith_types:
      | [numios, ~, ~, ~, current_types] = swreg_maskcheck(gcb);
      | % blk = gcb;
      | % mode = get_param(blk, 'mode');
      | % current_types = eval(get_param(blk, 'arith_types'));
      | % numios = length(current_types);
      | % if (strcmp(mode, 'one value') || strcmp(mode, 'fields of equal size')) && (length(current_types) > 1),
      | %     error('Only one type may be specified for this mode.');
      | % elseif strcmp(mode, 'fields of arbitrary size')
      | %     current_names = textscan(strtrim(strrep(strrep(get_param(blk, 'names'), ']', ''), '[', '')), '%s');
      | %     current_names = current_names{1};
      | %     numios = length(current_names);
      | %     if length(current_types) ~= numios,
      | %         error('%d field names specified, but %d types?', numios, length(current_types));
      | %     end
      | % end
      | problem = 0;
      | for ctr = 1 : numios,
      |     t = current_types(ctr);
      |     if (t < 0) || (t > 2),
      |         problem = t;
      |         ctr = numios + 1;
      |     end
      | end
      | if problem ~= 0,
      |     error('Type cannot be %i, must be 0, 1 or 2.', problem);
      | end
      mask Callback bin_pts:
      | swreg_maskcheck(gcb);
      | % blk = gcb;
      | % mode = get_param(blk, 'mode');
      | % current_bins = eval(get_param(blk, 'bin_pts'));
      | % if (strcmp(mode, 'one value') || strcmp(mode, 'fields of equal size')) && (length(current_bins) > 1),
      | %     error('Only one binary pt may be specified for this mode.');
      | % elseif strcmp(mode, 'fields of arbitrary size')
      | %     current_names = textscan(strtrim(strrep(strrep(get_param(blk, 'names'), ']', ''), '[', '')), '%s');
      | %     current_names = current_names{1};
      | %     numios = length(current_names);
      | %     if length(current_bins) ~= numios,
      | %         error('%d field names specified, but %d binary pts?', numios, length(current_bins));
      | %     end
      | % end
  snapshot : Subsystem  Tag=casper:snapshot  AncestorBlock=casper_library_scopes/snapshot  mask(snapshot){storage=bram, dram_dimm=1, dram_clock=200, nsamples=11, data_width=16, offset=off, circap=off, value=off, use_dsp48=on}
      mask prompts: storage "Storage medium"; dram_dimm "DRAM dimm"; dram_clock "DRAM clock rate"; nsamples "Number of Samples (2^?)"; data_width "Data width"; offset "Start delay support"; circap "Circular capture support"; value "Extra value capture support"; use_dsp48 "Use DSP48s to implement counters"
      mask help:
      | Standard snap block, but with the following optional extras;
      |  1) Optionally delay the fabric trigger by a user-specified number of valids.
      |  2) Capture continuously after a trigger until a stop pulse is received. Data is captured into BRAM continuously, with old data being overwritten until a stop command is received. Then stop capturing when memory is filled. This enables you to get some data before and some data after the stop pulse. Use the 'tr_en_cnt' register to determine where you are in your vector. 'Addr' register's MSb now indicates 'busy capturing'.
      |  3) Optionally capture a value on an input port to a register at the same time as the first data sample.
      |  4) Implement counters using DSP48Es to save resources.
      mask init: same as qdrdac_newphscrct/octoscope/snapshot
      mask TypeOptions storage: bram | dram
      mask Callback storage: snapshot_callback();
      mask TypeOptions dram_dimm: 1 | 2 | 3 | 4
      mask TypeOptions dram_clock: 200 | 250 | 266 | 300 | 333
      mask TypeOptions data_width: 8 | 16 | 32 | 64 | 128
  uint16_{0..7} (8 alike) : xbsIndex_r4/Reinterpret  force_arith_type=on  arith_type=Unsigned  force_bin_pt=on  bin_pt=0  block_type=reinterpret
  svdata : Outport
  wires:
  In6/1 -> uint16_5/1
  uint16_7/1 -> Mux/9
  uint16_6/1 -> Mux/8
  uint16_5/1 -> Mux/7
  uint16_4/1 -> Mux/6
  uint16_3/1 -> Mux/5
  uint16_2/1 -> Mux/4
  uint16_1/1 -> Mux/3
  uint16_0/1 -> Mux/2
  In8/1 -> uint16_7/1
  In7/1 -> uint16_6/1
  In5/1 -> uint16_4/1
  In4/1 -> uint16_3/1
  In3/1 -> uint16_2/1
  In2/1 -> uint16_1/1
  In1/1 -> uint16_0/1
  inputsel/1(in_reg) -> b3_0_/1
  b3_0_/1 -> Mux/1
  Constant3/1 -> inputsel/1(sim_1)
  Mux/1 -> snapshot/1(din), svdata/1
  Constant/1 -> snapshot/3(trig), snapshot/2(we)

== system qdrdac_newphscrct/scope_a ==
  In1 : Inport
  In2 : Inport  Port=2
  In3 : Inport  Port=3
  In4 : Inport  Port=4
  sync : Inport  Port=5
  Disregard Subsystem : xbsIndex_r4/Disregard Subsystem  Tag=discardX  block_type=disregard
  Gateway Out{1..9} (9 alike) : xbsIndex_r4/Gateway Out  inherit_from_input=off  hdl_port=on  timing_constraint=None  locs_specified=off  LOCs={}  UseAsDAC=off  DACChannel='1'  block_type=gatewayout
  c_to_ri{5..8} (4 alike) : casper_library_misc/c_to_ri  n_bits=18  bin_pt=16
      settings: AttributesFormatString=18_16 r/i
  pfbscope : Scope  NumInputPorts=9
      settings: YMin=-5~-5~-5~-5~-5~-5~-5~-5~-5  YMax=5~5~5~5~5~5~5~5~5  SaveName=pfboutput
  wires:
  Gateway Out7/1 -> pfbscope/4
  In1/1 -> c_to_ri5/1
  Gateway Out4/1 -> pfbscope/1
  c_to_ri8/2 -> Gateway Out8/1
  In4/1 -> c_to_ri8/1
  c_to_ri5/1 -> Gateway Out4/1
  c_to_ri6/1 -> Gateway Out6/1
  Gateway Out2/1 -> pfbscope/6
  c_to_ri8/1 -> Gateway Out3/1
  Gateway Out6/1 -> pfbscope/3
  c_to_ri7/2 -> Gateway Out2/1
  Gateway Out3/1 -> pfbscope/7
  Gateway Out8/1 -> pfbscope/8
  Gateway Out5/1 -> pfbscope/2
  c_to_ri5/2 -> Gateway Out5/1
  c_to_ri6/2 -> Gateway Out7/1
  In2/1 -> c_to_ri6/1
  Gateway Out1/1 -> pfbscope/5
  In3/1 -> c_to_ri7/1
  c_to_ri7/1 -> Gateway Out1/1
  Gateway Out9/1 -> pfbscope/9
  sync/1 -> Gateway Out9/1

== system qdrdac_newphscrct/scope_a1 ==
  In1 : Inport
  In2 : Inport  Port=2
  In3 : Inport  Port=3
  In4 : Inport  Port=4
  sync : Inport  Port=5
  Disregard Subsystem : xbsIndex_r4/Disregard Subsystem  Tag=discardX  block_type=disregard
  Gateway Out{1..9} (9 alike) : xbsIndex_r4/Gateway Out  inherit_from_input=off  hdl_port=on  timing_constraint=None  locs_specified=off  LOCs={}  UseAsDAC=off  DACChannel='1'  block_type=gatewayout
  c_to_ri{5..8} (4 alike) : casper_library_misc/c_to_ri  n_bits=18  bin_pt=16
      settings: AttributesFormatString=18_16 r/i
  pfbscope : Scope  NumInputPorts=9
      settings: YMin=-5~-5~-5~-5~-5~-5~-5~-5~-5  YMax=5~5~5~5~5~5~5~5~5  SaveName=fftoutput
  wires:
  Gateway Out7/1 -> pfbscope/4
  In1/1 -> c_to_ri5/1
  Gateway Out4/1 -> pfbscope/1
  c_to_ri8/2 -> Gateway Out8/1
  In4/1 -> c_to_ri8/1
  c_to_ri5/1 -> Gateway Out4/1
  c_to_ri6/1 -> Gateway Out6/1
  Gateway Out2/1 -> pfbscope/6
  c_to_ri8/1 -> Gateway Out3/1
  Gateway Out6/1 -> pfbscope/3
  c_to_ri7/2 -> Gateway Out2/1
  Gateway Out3/1 -> pfbscope/7
  Gateway Out8/1 -> pfbscope/8
  Gateway Out5/1 -> pfbscope/2
  c_to_ri5/2 -> Gateway Out5/1
  c_to_ri6/2 -> Gateway Out7/1
  In2/1 -> c_to_ri6/1
  Gateway Out1/1 -> pfbscope/5
  In3/1 -> c_to_ri7/1
  c_to_ri7/1 -> Gateway Out1/1
  Gateway Out9/1 -> pfbscope/9
  sync/1 -> Gateway Out9/1

== system qdrdac_newphscrct/scope_a2 ==
  In1 : Inport
  In2 : Inport  Port=2
  In3 : Inport  Port=3
  In4 : Inport  Port=4
  sync : Inport  Port=5
  Disregard Subsystem : xbsIndex_r4/Disregard Subsystem  Tag=discardX  block_type=disregard
  Gateway Out{1..9} (9 alike) : xbsIndex_r4/Gateway Out  inherit_from_input=off  hdl_port=on  timing_constraint=None  locs_specified=off  LOCs={}  UseAsDAC=off  DACChannel='1'  block_type=gatewayout
  c_to_ri{5..8} (4 alike) : casper_library_misc/c_to_ri  n_bits=18  bin_pt=16
      settings: AttributesFormatString=18_16 r/i
  pfbscope22 : Scope  NumInputPorts=9
      settings: YMin=-5~-5~-5~-5~-5~-5~-5~-5~-5  YMax=5~5~5~5~5~5~5~5~5  SaveName=fftoutput2
  wires:
  Gateway Out7/1 -> pfbscope22/4
  In1/1 -> c_to_ri5/1
  Gateway Out4/1 -> pfbscope22/1
  c_to_ri8/2 -> Gateway Out8/1
  In4/1 -> c_to_ri8/1
  c_to_ri5/1 -> Gateway Out4/1
  c_to_ri6/1 -> Gateway Out6/1
  Gateway Out2/1 -> pfbscope22/6
  c_to_ri8/1 -> Gateway Out3/1
  Gateway Out6/1 -> pfbscope22/3
  c_to_ri7/2 -> Gateway Out2/1
  Gateway Out3/1 -> pfbscope22/7
  Gateway Out8/1 -> pfbscope22/8
  Gateway Out5/1 -> pfbscope22/2
  c_to_ri5/2 -> Gateway Out5/1
  c_to_ri6/2 -> Gateway Out7/1
  In2/1 -> c_to_ri6/1
  Gateway Out1/1 -> pfbscope22/5
  In3/1 -> c_to_ri7/1
  c_to_ri7/1 -> Gateway Out1/1
  Gateway Out9/1 -> pfbscope22/9
  sync/1 -> Gateway Out9/1

== system qdrdac_newphscrct/sw_timestamp ==
  sim_1 : Inport
  io_delay : xbsIndex_r4/Delay  rst=off  infoeditControl=Selection of Reset will increase slice count due to use of real FFs and instead of SRLs  en=off  latency=0  dbl_ovrd=off  reg_retiming=on  block_type=delay
  qdrdac_sw_timestamp_user_data_out : xbsIndex_r4/Gateway In  gui_display_data_type=Fixed-point  arith_type=Unsigned  n_bits=32  bin_pt=0  preci_type=Single  exp_width=8  frac_width=24  quantization="Round  (unbiased: +/- Inf)"  overflow=Saturate  period=1  dbl_ovrd=off  timing_constraint=None  locs_specified=off  LOCs={}  UseAsADC=off  ADCChannel='1'  inherit_from_input=off  hdl_port=on  block_type=gatewayin
  reint1 : xbsIndex_r4/Reinterpret  force_arith_type=on  arith_type=Unsigned  force_bin_pt=on  bin_pt=0  block_type=reinterpret
  slice_reg : xbsIndex_r4/Slice  nbits=32  boolean_output=off  mode=Lower Bit Location + Width  bit1=0  base1=MSB of Input  bit0=0  base0=LSB of Input  dbl_ovrd=off  block_type=slice
  in_reg : Outport
  wires:
  qdrdac_sw_timestamp_user_data_out/1 -> io_delay/1
  sim_1/1 -> qdrdac_sw_timestamp_user_data_out/1
  io_delay/1 -> slice_reg/1
  slice_reg/1 -> reint1/1
  reint1/1 -> in_reg/1

== system qdrdac_newphscrct/sw_timestamp2 ==
  sim_1 : Inport
  io_delay : xbsIndex_r4/Delay  rst=off  infoeditControl=Selection of Reset will increase slice count due to use of real FFs and instead of SRLs  en=off  latency=0  dbl_ovrd=off  reg_retiming=on  block_type=delay
  qdrdac_sw_timestamp2_user_data_out : xbsIndex_r4/Gateway In  gui_display_data_type=Fixed-point  arith_type=Unsigned  n_bits=32  bin_pt=0  preci_type=Single  exp_width=8  frac_width=24  quantization="Round  (unbiased: +/- Inf)"  overflow=Saturate  period=1  dbl_ovrd=off  timing_constraint=None  locs_specified=off  LOCs={}  UseAsADC=off  ADCChannel='1'  inherit_from_input=off  hdl_port=on  block_type=gatewayin
  reint1 : xbsIndex_r4/Reinterpret  force_arith_type=on  arith_type=Unsigned  force_bin_pt=on  bin_pt=0  block_type=reinterpret
  slice_reg : xbsIndex_r4/Slice  nbits=32  boolean_output=off  mode=Lower Bit Location + Width  bit1=0  base1=MSB of Input  bit0=0  base0=LSB of Input  dbl_ovrd=off  block_type=slice
  in_reg : Outport
  wires:
  qdrdac_sw_timestamp2_user_data_out/1 -> io_delay/1
  sim_1/1 -> qdrdac_sw_timestamp2_user_data_out/1
  io_delay/1 -> slice_reg/1
  slice_reg/1 -> reint1/1
  reint1/1 -> in_reg/1
